simulink model "phiPID"  (R2019a)
settings: Solver=VariableStepAuto  StartTime=0.0  StopTime=10  RelTol=1e-3
values from neighbouring files (symbols this model uses):
  a = [A2(1) A1(1) A2(2) A1(2) A2(3)]    [SystemID.m]    (also in animation.m = 2)
  b = [B2(1) B2(2) B1(1) B1(2) B2(3)]    [SystemID.m]    (also in animation.m = 5)
undefined symbols (not defined in the file or in its folder): DiscIntNeverNeededParam
libraries: simulink x1
settings Model: Creator=free9  LastModifiedBy=free9

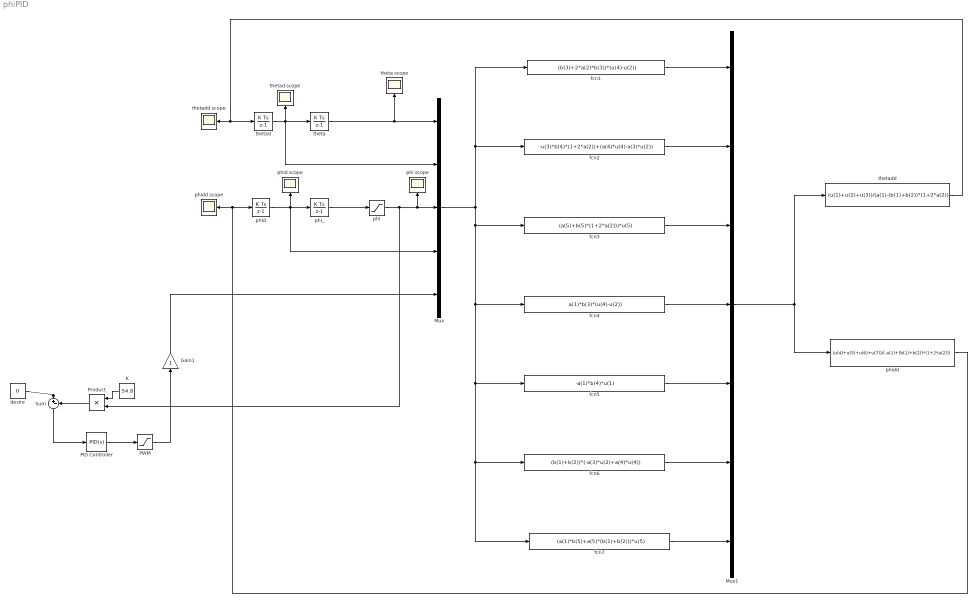
== system phiPID ==
  Gain1 : Gain
  K : Constant  Value=54.8
  Mux : Mux  Inputs=5
  Mux1 : Mux  Inputs=7
  PID Controller : simulink/Continuous/PID Controller  Controller=PID  Form=Parallel  TimeDomain=Continuous-time  SampleTime=-1  IntegratorMethod=Forward Euler  FilterMethod=Forward Euler  ControllerParametersSource=internal  P=24  I=180  D=0.8  UseFilter=on  N=1000  TunerSelectOption=Transfer Function Based (PID Tuner App)  InitialConditionSource=internal  InitialConditionForIntegrator=0  InitialConditionForFilter=0  DifferentiatorICPrevScaledInput=0  ExternalReset=none  TrackingMode=off  Kt=1  LimitOutput=off  UpperSaturationLimit=inf  LowerSaturationLimit=-inf  LinearizeAsGain=on  AntiWindupMode=none  Kb=1  POutMin=[]  POutMax=[]  IOutMin=[]  IOutMax=[]  DOutMin=[]  DOutMax=[]  NOutMin=[]  NOutMax=[]  SumOutMin=[]  SumOutMax=[]  SaturationOutMin=[]  SaturationOutMax=[]  PParamMin=[]  PParamMax=[]  IParamMin=[]  IParamMax=[]  DParamMin=[]  DParamMax=[]  NParamMin=[]  NParamMax=[]  KbParamMin=[]  KbParamMax=[]  KtParamMin=[]  KtParamMax=[]  KbOutMin=[]  KbOutMax=[]  KtOutMin=[]  KtOutMax=[]  IntegratorOutMin=[]  IntegratorOutMax=[]  FilterOutMin=[]  FilterOutMax=[]  SumI1OutMin=[]  SumI1OutMax=[]  SumI2OutMin=[]  SumI2OutMax=[]  SumI3OutMin=[]  SumI3OutMax=[]  SumI4OutMin=[]  SumI4OutMax=[]  SumDOutMin=[]  SumDOutMax=[]  DifferentiatorOutMin=[]  DifferentiatorOutMax=[]  FilterDiffOutCoefMin=[]  FilterDiffOutCoefMax=[]  ReciprocalOutMin=[]  ReciprocalOutMax=[]  SumDenOutMin=[]  SumDenOutMax=[]  SumNumOutMin=[]  SumNumOutMax=[]  DivideOutMin=[]  DivideOutMax=[]  IntegratorContinuousStateAttributes=''  IntegratorStateMustResolveToSignalObject=off  IntegratorRTWStateStorageClass=Auto  FilterContinuousStateAttributes=''  FilterStateMustResolveToSignalObject=off  FilterRTWStateStorageClass=Auto  ParallelPVariant=InternalParameters  IdealPVariant=Disabled  IVariant=InternalParameters  DVariant=InternalParameters  IntegratorVariant=Continuous  SatVariant=Disabled  AWVariant=Passthrough  PCopyVariant=Disabled  TRVariant=Disabled  FdbkBlocksVariant=Forward  IdealPFdbkVariant=Disabled  SatFdbkVariant=Disabled  DerivativeFilterVariant=ContFilter  NVariant=InternalParameters  NCopyVariant=Disabled  FilterICVariant=InternalICsFilter  IntegratorICVariant=InternalICs  ExternalResetVariant=Disabled  TRSumVariant=Passthrough  SumFdbkVariant=Disabled  SumVariant=Sum_PID
  PWM : Saturate  UpperLimit=255  LowerLimit=-255
  Product : Product
  Sum : Sum  Inputs=|+-
  desire : Constant  Value=0
  "fcn1 " : Fcn  Expr=(b(3)+2*a(2)*b(3))*(u(4)-u(2))
  fcn2 : Fcn  Expr=-u(3)*b(4)*(1+2*a(2))+(a(4)*u(4)-a(3)*u(2))
  "fcn3 " : Fcn  Expr=(a(5)+b(5)*(1+2*a(2)))*u(5)
  fcn4 : Fcn  Expr=a(1)*b(3)*(u(4)-u(2))
  fcn5 : Fcn  Expr=-a(1)*b(4)*u(1)
  fcn6 : Fcn  Expr=(b(1)+b(2))*(-a(3)*u(2)+a(4)*u(4))
  fcn7 : Fcn  Expr=(a(1)*b(5)+a(5)*(b(1)+b(2)))*u(5)
  phi : Saturate  UpperLimit=1.6  LowerLimit=-1.6
  "phi scope " : Scope
  phi_ : DiscreteIntegrator  InitialCondition=pi/180  SampleTime=0.001  ICPrevOutput=DiscIntNeverNeededParam  ICPrevScaledInput=DiscIntNeverNeededParam
  phid : DiscreteIntegrator  SampleTime=0.001  ICPrevOutput=DiscIntNeverNeededParam  ICPrevScaledInput=DiscIntNeverNeededParam
  "phid scope " : Scope
  phidd : Fcn  Expr=(u(4)+u(5)+u(6)+u(7))/(-a(1)+(b(1)+b(2))*(1+2*a(2)))
  "phidd scope " : Scope
  theta : DiscreteIntegrator  SampleTime=0.001  ICPrevOutput=DiscIntNeverNeededParam  ICPrevScaledInput=DiscIntNeverNeededParam
  theta scope : Scope
  thetad : DiscreteIntegrator  SampleTime=0.001  ICPrevOutput=DiscIntNeverNeededParam  ICPrevScaledInput=DiscIntNeverNeededParam
  "thetad scope " : Scope
  thetadd : Fcn  Expr=(u(1)+u(2)+u(3))/(a(1)-(b(1)+b(2))*(1+2*a(2)))
  "thetadd scope " : Scope
  wires:
  Product/1 -> Sum/2
  PWM/1 -> Gain1/1
  Sum/1 -> PID Controller/1
  theta/1 -> theta scope/1, Mux/1
  Mux1/1 -> thetadd/1, phidd/1
  PID Controller/1 -> PWM/1
  Mux/1 -> "fcn3 "/1, fcn4/1, fcn7/1, fcn6/1, fcn5/1, "fcn1 "/1, fcn2/1
  desire/1 -> Sum/1
  phi_/1 -> phi/1
  "fcn1 "/1 -> Mux1/1
  fcn7/1 -> Mux1/7
  thetadd/1 -> thetad/1, "thetadd scope "/1
  fcn5/1 -> Mux1/5
  phidd/1 -> "phidd scope "/1, phid/1
  thetad/1 -> "thetad scope "/1, theta/1, Mux/2
  phid/1 -> Mux/4, phi_/1, "phid scope "/1
  K/1 -> Product/1
  fcn6/1 -> Mux1/6
  fcn4/1 -> Mux1/4
  "fcn3 "/1 -> Mux1/3
  phi/1 -> Mux/3, "phi scope "/1, Product/2
  fcn2/1 -> Mux1/2
  Gain1/1 -> Mux/5
